simulink subsystem "mesh_assembly"  (R2021a)
settings: Solver=VariableStepAuto  StartTime=0.0  StopTime=10.0  RelTol=1e-3
undefined symbols (not defined in the file): dnm, knm, X, Y, Z
libraries: sm_lib x110, mesh_assembly_library x15
(part 1 of 4)
settings Model: DefaultTestHarness=mechanics_model_measure_transforms  Creator=Daniel Adejumo  LastModifiedBy=Daniel Adejumo

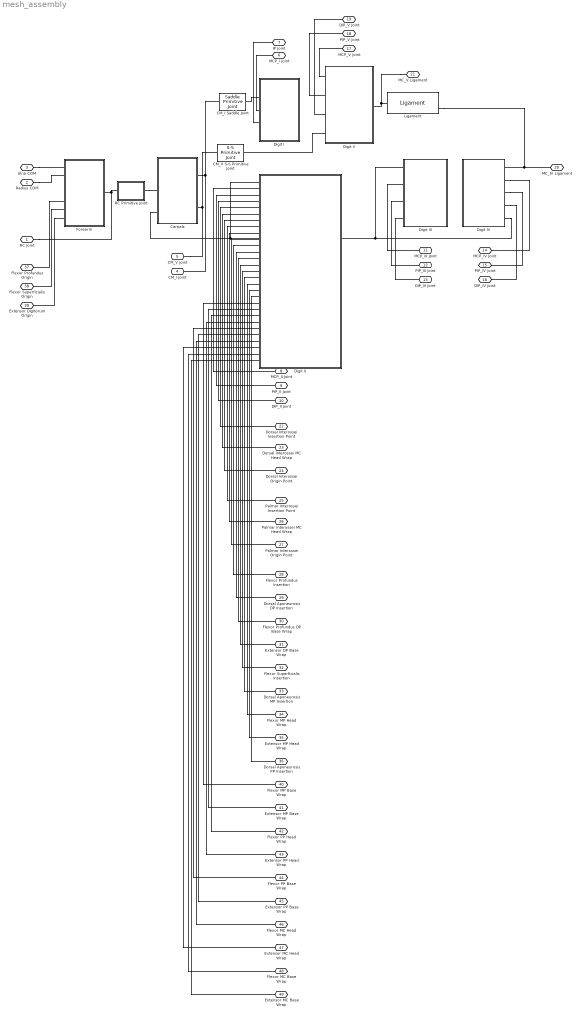
== system mesh_assembly ==
  CM_I Saddle Joint : mesh_assembly_library/Saddle Primitive Joint  stiffness=0  damping=0  x_limits=[-90 90]  y_limits=[-90 90]  z_limits=[-90 90]  x_initial_position=0  y_initial_position=0  z_initial_position=0  centre_block_dim=knm.carpals.cm_i_joint_centre_block_dim  centre_block_density=0  thickness=viz.carpals.cm_1_joint.thickness  x_radius=viz.carpals.cm_1_joint.x_radius  x_length=viz.carpals.cm_1_joint.x_length  x_color=viz.carpals.cm_1_joint.x_color  x_opacity=viz.carpals.cm_1_joint.x_opacity  y_radius=viz.carpals.cm_1_joint.y_radius  y_length=viz.carpals.cm_1_joint.y_length  y_color=viz.carpals.cm_1_joint.y_color  y_opacity=viz.carpals.cm_1_joint.y_opacity  z_radius=viz.carpals.cm_1_joint.z_radius  z_length=viz.carpals.cm_1_joint.z_length  z_color=viz.carpals.cm_1_joint.z_color  z_opacity=viz.carpals.cm_1_joint.z_opacity
  CM_V S-S Primitive Joint : mesh_assembly_library/S-S Primitive Joint  stiffness=0  damping=0  x_limits=[-90 90]  y_limits=[-90 90]  x_initial_position=0  y_initial_position=0  radius=viz.carpals.cm_v_joint.radius  color=viz.carpals.cm_v_joint.color  opacity=viz.carpals.cm_v_joint.opacity
  Carpals : Subsystem
  Digit I : Subsystem
  Digit II : Subsystem
  Digit III : Subsystem
  Digit IV : Subsystem
  Digit V : Subsystem
  Forearm : Subsystem
  Ligament : mesh_assembly_library/Ligament  length=knm.d5.metacarpal_head_ligament.length  width=knm.d5.metacarpal_head_ligament.width  thickness=knm.d5.metacarpal_head_ligament.thickness  tension_stiffness=35E3  tension_damping_coefficient=100  transition_region_width=1e-3  density=800  damping_coefficient=0.2
  RC Primitive Joint : Subsystem  AncestorBlock=mechanics_model_library/S-S Primitive Joint  mask{stiffness=0, damping=0, x_limits=[-90 90], y_limits=[-90 90], x_initial_position=0, y_initial_position=0, thickness=viz.forearm.rc_joint.thickness, x_radius=viz.forearm.rc_joint.x_radius, x_length=viz.forearm.rc_joint.x_length, x_color=viz.forearm.rc_joint.x_color, x_opacity=viz.forearm.rc_joint.x_opacity, y_radius=viz.forearm.rc_joint.y_radius, y_length=viz.forearm.rc_joint.y_length, y_color=viz.forearm.rc_joint.y_color, y_opacity=viz.forearm.rc_joint.y_opacity}
      mask prompts: x_limits "X Limits"; y_limits "Y Limits"; x_initial_position "X Initial Position"; y_initial_position "Y Initial Position"; thickness "Thickness [m]"; x_radius "X Radius [m]"; x_length "X Length [m]"; x_color "X Color (RGB - Range [0, 1])"; x_opacity "X Opacity (Range [0, 1])"; y_radius "Y Radius [m]"; y_length "Y Length [m]"; y_color "Y Color (RGB - Range [0, 1])"; y_opacity "Y Opacity (Range [0, 1])"
      mask DialogControl DescGroupVar Prompt: Radiocarpal Primitive Joint
      mask DialogControl DescTextVar Prompt: Primitive representation of the radiocarpal joint using a universal joint. This is found at the Radiocarpal joint.
      mask DialogControl Container4 Prompt: Mechanics
      mask DialogControl Container6 Prompt: Visualization
      mask DialogControl Container7 Prompt: X Axis
      mask DialogControl Container8 Prompt: Y Axis
  RC Joint : PMIOPort  Side=Left
  Radius COM : PMIOPort  Port=2  Side=Left
  Ulna COM : PMIOPort  Port=3  Side=Left
  CM_I Joint : PMIOPort  Port=4  Side=Left
  CM_V Joint : PMIOPort  Port=5  Side=Left
  MCP_I Joint : PMIOPort  Port=6  Side=Left
  IP Joint : PMIOPort  Port=7  Side=Left
  MCP_II Joint : PMIOPort  Port=8  Side=Left
  PIP_II Joint : PMIOPort  Port=9  Side=Left
  DIP_II Joint : PMIOPort  Port=10  Side=Left
  MCP_III Joint : PMIOPort  Port=11  Side=Left
  PIP_III Joint : PMIOPort  Port=12  Side=Left
  DIP_III Joint : PMIOPort  Port=13  Side=Left
  MCP_IV Joint : PMIOPort  Port=14  Side=Left
  PIP_IV Joint : PMIOPort  Port=15  Side=Left
  DIP_IV Joint : PMIOPort  Port=16  Side=Left
  MCP_V Joint : PMIOPort  Port=17  Side=Left
  PIP_V Joint : PMIOPort  Port=18  Side=Left
  DIP_V Joint : PMIOPort  Port=19  Side=Left
  MC_IV Ligament : PMIOPort  Port=20  Side=Right
  MC_V Ligament : PMIOPort  Port=21  Side=Right
  Dorsal Interossei Insertion Point : PMIOPort  Port=22  Side=Left
  Dorsal Interossei MC Head Wrap : PMIOPort  Port=23  Side=Left
  Dorsal Interossei Origin Point : PMIOPort  Port=24  Side=Left
  Palmar Interossei Insertion Point : PMIOPort  Port=25  Side=Left
  Palmar Interossei MC Head Wrap : PMIOPort  Port=26  Side=Left
  Palmar Interossei Origin Point : PMIOPort  Port=27  Side=Left
  Flexor Profundus Insertion : PMIOPort  Port=28  Side=Left
  Dorsal Aponeurosis DP Insertion : PMIOPort  Port=29  Side=Left
  Flexor Profundus DP Base Wrap : PMIOPort  Port=30  Side=Left
  Extensor DP Base Wrap : PMIOPort  Port=31  Side=Left
  Flexor Superficialis Insertion : PMIOPort  Port=32  Side=Left
  Dorsal Aponeurosis MP Insertion : PMIOPort  Port=33  Side=Left
  Flexor MP Head Wrap : PMIOPort  Port=34  Side=Left
  Extensor MP Head Wrap : PMIOPort  Port=35  Side=Left
  Dorsal Aponeurosis PP Insertion : PMIOPort  Port=36  Side=Left
  Flexor Profundus Origin : PMIOPort  Port=37  Side=Left
  Flexor Superficialis Origin : PMIOPort  Port=38  Side=Left
  Extensor Digitorum Origin : PMIOPort  Port=39  Side=Left
  Flexor MP Base Wrap : PMIOPort  Port=40  Side=Left
  Extensor MP Base Wrap : PMIOPort  Port=41  Side=Left
  Flexor PP Head Wrap : PMIOPort  Port=42  Side=Left
  Extensor PP Head Wrap : PMIOPort  Port=43  Side=Left
  Flexor PP Base Wrap : PMIOPort  Port=44  Side=Left
  Extensor PP Base Wrap : PMIOPort  Port=45  Side=Left
  Flexor MC Head Wrap : PMIOPort  Port=46  Side=Left
  Extensor MC Head Wrap : PMIOPort  Port=47  Side=Left
  Flexor MC Base Wrap : PMIOPort  Port=48  Side=Left
  Extensor MC Base Wrap : PMIOPort  Port=49  Side=Left
  connections:
  RC Primitive Joint/LConn1 -- Forearm/RConn1 -- RC Joint/RConn1
  Digit IV/LConn5 -- Digit III/LConn1 -- Digit II/LConn1 -- Carpals/LConn3
  CM_I Joint/RConn1 -- Carpals/RConn1 -- CM_I Saddle Joint/LConn1
  MC_V Ligament/RConn1 -- Ligament/LConn1 -- Digit V/RConn1
  CM_V Joint/RConn1 -- Carpals/RConn2 -- CM_V S-S Primitive Joint/LConn1
  MC_IV Ligament/RConn1 -- Ligament/RConn1 -- Digit IV/LConn1
  Digit V/LConn4 -- CM_V S-S Primitive Joint/RConn1
  Digit I/LConn2 -- CM_I Saddle Joint/RConn1
  Radius COM/RConn1 -- Forearm/LConn2
  Ulna COM/RConn1 -- Forearm/LConn1
  MCP_I Joint/RConn1 -- Digit I/LConn3
  IP Joint/RConn1 -- Digit I/LConn4
  Digit II/LConn2 -- MCP_II Joint/RConn1
  Digit II/LConn3 -- PIP_II Joint/RConn1
  Digit II/LConn4 -- DIP_II Joint/RConn1
  Digit III/LConn4 -- DIP_III Joint/RConn1
  Digit III/LConn3 -- PIP_III Joint/RConn1
  Digit III/LConn2 -- MCP_III Joint/RConn1
  Digit IV/LConn2 -- MCP_IV Joint/RConn1
  Digit IV/LConn3 -- PIP_IV Joint/RConn1
  Digit IV/LConn4 -- DIP_IV Joint/RConn1
  PIP_V Joint/RConn1 -- Digit V/LConn2
  Digit V/LConn3 -- DIP_V Joint/RConn1
  MCP_V Joint/RConn1 -- Digit V/LConn1
  RC Primitive Joint/RConn1 -- Carpals/LConn2
  Digit II/LConn5 -- Dorsal Interossei Insertion Point/RConn1
  Digit II/LConn6 -- Dorsal Interossei MC Head Wrap/RConn1
  Digit II/LConn7 -- Dorsal Interossei Origin Point/RConn1
  Digit II/LConn8 -- Palmar Interossei Insertion Point/RConn1
  Digit II/LConn9 -- Palmar Interossei MC Head Wrap/RConn1
  Digit II/LConn10 -- Palmar Interossei Origin Point/RConn1
  Digit II/LConn11 -- Flexor Profundus Insertion/RConn1
  Digit II/LConn12 -- Dorsal Aponeurosis DP Insertion/RConn1
  Digit II/LConn13 -- Flexor Profundus DP Base Wrap/RConn1
  Digit II/LConn14 -- Extensor DP Base Wrap/RConn1
  Digit II/LConn15 -- Flexor Superficialis Insertion/RConn1
  Digit II/LConn16 -- Dorsal Aponeurosis MP Insertion/RConn1
  Digit II/LConn17 -- Flexor MP Head Wrap/RConn1
  Digit II/LConn18 -- Extensor MP Head Wrap/RConn1
  Digit II/LConn19 -- Dorsal Aponeurosis PP Insertion/RConn1
  Forearm/LConn5 -- Flexor Profundus Origin/RConn1
  Forearm/LConn6 -- Flexor Superficialis Origin/RConn1
  Forearm/LConn7 -- Extensor Digitorum Origin/RConn1
  Digit II/LConn20 -- Flexor MP Base Wrap/RConn1
  Digit II/LConn21 -- Extensor MP Base Wrap/RConn1
  Digit II/LConn22 -- Flexor PP Head Wrap/RConn1
  Digit II/LConn23 -- Extensor PP Head Wrap/RConn1
  Digit II/LConn24 -- Flexor PP Base Wrap/RConn1
  Digit II/LConn25 -- Extensor PP Base Wrap/RConn1
  Digit II/LConn26 -- Flexor MC Head Wrap/RConn1
  Digit II/LConn27 -- Extensor MC Head Wrap/RConn1
  Digit II/LConn28 -- Flexor MC Base Wrap/RConn1
  Digit II/LConn29 -- Extensor MC Base Wrap/RConn1

== system mesh_assembly/Carpals ==
  CM_I Joint Transform : sm_lib/Frames and Transforms/Rigid Transform  TranslationMethod=Cartesian  TranslationStandardOffset=0  TranslationLengthUnit=m  TranslationStandardAxis=+Z  TranslationCartesianOffset=knm.carpals.cm_i_joint_transform(1, :)  TranslationROffset=0  TranslationROffsetUnits=m  TranslationZOffset=0  TranslationZOffsetUnits=m  TranslationThetaOffset=0  TranslationThetaOffsetUnits=deg  RotationMethod=RotationSequence  RotationAngleUnits=deg  RotationStandardAxis=+Z  RotationAngle=0.0  RotationArbitraryAxis=[0 0 1]  FollAlignAxisA=+X  BaseAlignAxisA=+Y  FollAlignAxisB=+Y  BaseAlignAxisB=+Z  RotationSequenceAxes=FollowerAxes  RotationSequence=XYZ  RotationSequenceAngles=knm.carpals.cm_i_joint_transform(2, :)  RotationSequenceAnglesUnits=deg  RotationMatrix=[1 0 0; 0 1 0; 0 0 1]
  CM_V Joint Transform : sm_lib/Frames and Transforms/Rigid Transform  TranslationMethod=Cartesian  TranslationStandardOffset=0  TranslationLengthUnit=m  TranslationStandardAxis=+Z  TranslationCartesianOffset=knm.carpals.cm_v_joint_transform(1, :)  TranslationROffset=0  TranslationROffsetUnits=m  TranslationZOffset=0  TranslationZOffsetUnits=m  TranslationThetaOffset=0  TranslationThetaOffsetUnits=deg  RotationMethod=RotationSequence  RotationAngleUnits=deg  RotationStandardAxis=+Z  RotationAngle=0.0  RotationArbitraryAxis=[0 0 1]  FollAlignAxisA=+X  BaseAlignAxisA=+Y  FollAlignAxisB=+Y  BaseAlignAxisB=+Z  RotationSequenceAxes=FollowerAxes  RotationSequence=XYZ  RotationSequenceAngles=knm.carpals.cm_v_joint_transform(2, :)  RotationSequenceAnglesUnits=deg  RotationMatrix=[1 0 0; 0 1 0; 0 0 1]
  Carpals : sm_lib/Body Elements/File Solid  ExtGeomFileName=C:\Users\Daniel Adejumo\Documents\MATLAB\DARM\Geometry Models and FEA\Models\Skeleton Scan\Right Hand\Carpals.obj  UnitType=Custom  ExtGeomFileUnits=mm  StepReaderType=HEX  ExportConvexHullGeometry=off  InertiaType=CalculateFromGeometry  Mass=1  MassUnits=kg  CenterOfMass=[0 0 0]  CenterOfMassUnits=m  MomentsOfInertia=[1 1 1]  MomentsOfInertiaUnits=kg*m^2  ProductsOfInertia=[0 0 0]  ProductsOfInertiaUnits=kg*m^2  BasedOnType=Density  Density=dnm.link_density  DensityUnits=kg/m^3  DoExposeReferenceFrame=on  SerializedFrames=<Frames><Frame><Id>Frame1</Id><Value><Name>COM</Name><Origin><Source>CenterOfMassFrame</Source><FeatureName></FeatureName></Origin><PrimaryAxis><DefinedDirection>+Z</DefinedDirection><Source>ReferenceFrame</Source><SourceDirection>-Z</SourceDirection><FeatureName></FeatureName></PrimaryAxis><SecondaryAxis><DefinedDirection>+X</DefinedDirection><Source>ReferenceFrame</Source><SourceDirection>-Y</SourceDirection><FeatureName></FeatureName></SecondaryAxis></Value></Frame></Frames>  GraphicType=FromGeometry  MarkerShape=Sphere  MarkerSize=10  GraphicVisPropType=SimpleVisualProperties  GraphicDiffuseColor=[0.5 0.5 0.5]  GraphicSpecularColor=[0.5 0.5 0.5 1.0]  GraphicAmbientColor=[0.15 0.15 0.15 1.0]  GraphicEmissiveColor=[0.0 0.0 0.0 1.0]  GraphicShininess=75  GraphicOpacity=1.0
  RC Joint Transform : sm_lib/Frames and Transforms/Rigid Transform  TranslationMethod=Cartesian  TranslationStandardOffset=0  TranslationLengthUnit=m  TranslationStandardAxis=+Z  TranslationCartesianOffset=knm.carpals.rc_joint_transform(1, :)  TranslationROffset=0  TranslationROffsetUnits=m  TranslationZOffset=0  TranslationZOffsetUnits=m  TranslationThetaOffset=0  TranslationThetaOffsetUnits=deg  RotationMethod=RotationSequence  RotationAngleUnits=deg  RotationStandardAxis=+Z  RotationAngle=0.0  RotationArbitraryAxis=[0 0 1]  FollAlignAxisA=+X  BaseAlignAxisA=+Y  FollAlignAxisB=+Y  BaseAlignAxisB=+Z  RotationSequenceAxes=FollowerAxes  RotationSequence=XYZ  RotationSequenceAngles=knm.carpals.rc_joint_transform(2, :)  RotationSequenceAnglesUnits=deg  RotationMatrix=[1 0 0; 0 1 0; 0 0 1]
  Carpals COM : PMIOPort  Side=Left
  RC Joint : PMIOPort  Port=2  Side=Left
  Carpals R : PMIOPort  Port=3  Side=Left
  CM_I Joint : PMIOPort  Port=4  Side=Right
  CM_V Joint : PMIOPort  Port=5  Side=Right
  connections:
  CM_V Joint/RConn1 -- CM_V Joint Transform/RConn1
  CM_I Joint/RConn1 -- CM_I Joint Transform/RConn1
  Carpals R/RConn1 -- Carpals/RConn1
  CM_I Joint Transform/LConn1 -- Carpals/LConn1 -- CM_V Joint Transform/LConn1 -- RC Joint Transform/LConn1 -- Carpals COM/RConn1
  RC Joint/RConn1 -- RC Joint Transform/RConn1

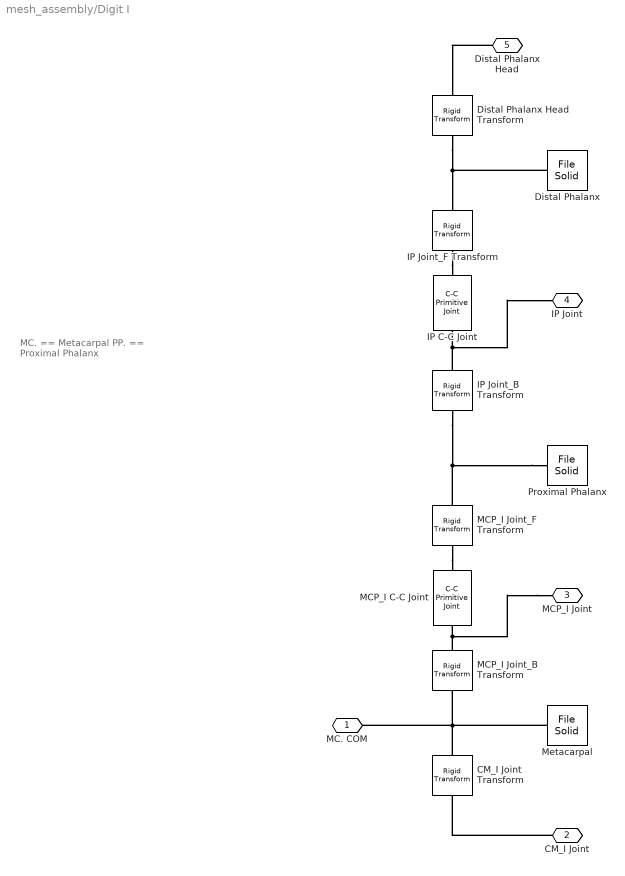
== system mesh_assembly/Digit I ==
  note: MC. == Metacarpal
      | PP. == Proximal Phalanx
  CM_I Joint Transform : sm_lib/Frames and Transforms/Rigid Transform  TranslationMethod=Cartesian  TranslationStandardOffset=0  TranslationLengthUnit=m  TranslationStandardAxis=+Z  TranslationCartesianOffset=knm.d1.metacarpal.cm_joint_transform(1, :)  TranslationROffset=0  TranslationROffsetUnits=m  TranslationZOffset=0  TranslationZOffsetUnits=m  TranslationThetaOffset=0  TranslationThetaOffsetUnits=deg  RotationMethod=RotationSequence  RotationAngleUnits=deg  RotationStandardAxis=+Z  RotationAngle=0.0  RotationArbitraryAxis=[0 0 1]  FollAlignAxisA=+X  BaseAlignAxisA=+Y  FollAlignAxisB=+Y  BaseAlignAxisB=+Z  RotationSequenceAxes=FollowerAxes  RotationSequence=XYZ  RotationSequenceAngles=knm.d1.metacarpal.cm_joint_transform(2, :)  RotationSequenceAnglesUnits=deg  RotationMatrix=[1 0 0; 0 1 0; 0 0 1]
  Distal Phalanx : sm_lib/Body Elements/File Solid  ExtGeomFileName=C:\Users\Daniel Adejumo\Documents\MATLAB\DARM\Geometry Models and FEA\Models\Skeleton Scan\Right Hand\Digit I\Distal Phalanx I.obj  UnitType=Custom  ExtGeomFileUnits=in  StepReaderType=HEX  ExportConvexHullGeometry=off  InertiaType=CalculateFromGeometry  Mass=1  MassUnits=kg  CenterOfMass=[0 0 0]  CenterOfMassUnits=m  MomentsOfInertia=[1 1 1]  MomentsOfInertiaUnits=kg*m^2  ProductsOfInertia=[0 0 0]  ProductsOfInertiaUnits=kg*m^2  BasedOnType=Density  Density=dnm.link_density  DensityUnits=kg/m^3  DoExposeReferenceFrame=on  SerializedFrames=<Frames><Frame><Id>Frame1</Id><Value><Name>COM</Name><Origin><Source>CenterOfMassFrame</Source><FeatureName></FeatureName></Origin><PrimaryAxis><DefinedDirection>+Z</DefinedDirection><Source>ReferenceFrame</Source><SourceDirection>-Z</SourceDirection><FeatureName></FeatureName></PrimaryAxis><SecondaryAxis><DefinedDirection>+X</DefinedDirection><Source>ReferenceFrame</Source><SourceDirection>+X</SourceDirection><FeatureName></FeatureName></SecondaryAxis></Value></Frame></Frames>  GraphicType=FromGeometry  MarkerShape=Sphere  MarkerSize=10  GraphicVisPropType=SimpleVisualProperties  GraphicDiffuseColor=[0.5 0.5 0.5]  GraphicSpecularColor=[0.5 0.5 0.5 1.0]  GraphicAmbientColor=[0.15 0.15 0.15 1.0]  GraphicEmissiveColor=[0.0 0.0 0.0 1.0]  GraphicShininess=75  GraphicOpacity=1.0
  Distal Phalanx Head Transform : sm_lib/Frames and Transforms/Rigid Transform  TranslationMethod=Cartesian  TranslationStandardOffset=0  TranslationLengthUnit=m  TranslationStandardAxis=+Z  TranslationCartesianOffset=knm.d1.distal_phalanx.head_transform(1, :)  TranslationROffset=0  TranslationROffsetUnits=m  TranslationZOffset=0  TranslationZOffsetUnits=m  TranslationThetaOffset=0  TranslationThetaOffsetUnits=deg  RotationMethod=RotationSequence  RotationAngleUnits=deg  RotationStandardAxis=+Z  RotationAngle=0.0  RotationArbitraryAxis=[0 0 1]  FollAlignAxisA=+X  BaseAlignAxisA=+Y  FollAlignAxisB=+Y  BaseAlignAxisB=+Z  RotationSequenceAxes=FollowerAxes  RotationSequence=XYZ  RotationSequenceAngles=knm.d1.distal_phalanx.head_transform(2, :)  RotationSequenceAnglesUnits=deg  RotationMatrix=[1 0 0; 0 1 0; 0 0 1]
  IP C-C Joint : mesh_assembly_library/C-C Primitive Joint  stiffness=0  damping=0  lower_limit=-90  upper_limit=90  initial_position=0  radius=viz.d1.ip_joint.radius  length=viz.d1.ip_joint.length  thickness=viz.d1.ip_joint.thickness  color=viz.d1.ip_joint.color  opacity=viz.d1.ip_joint.opacity
  IP Joint_B Transform : sm_lib/Frames and Transforms/Rigid Transform  TranslationMethod=Cartesian  TranslationStandardOffset=0  TranslationLengthUnit=m  TranslationStandardAxis=+Z  TranslationCartesianOffset=knm.d1.proximal_phalanx.ip_joint_transform(1, :)  TranslationROffset=0  TranslationROffsetUnits=m  TranslationZOffset=0  TranslationZOffsetUnits=m  TranslationThetaOffset=0  TranslationThetaOffsetUnits=deg  RotationMethod=RotationSequence  RotationAngleUnits=deg  RotationStandardAxis=+Z  RotationAngle=0.0  RotationArbitraryAxis=[0 0 1]  FollAlignAxisA=+X  BaseAlignAxisA=+Y  FollAlignAxisB=+Y  BaseAlignAxisB=+Z  RotationSequenceAxes=FollowerAxes  RotationSequence=XYZ  RotationSequenceAngles=knm.d1.proximal_phalanx.ip_joint_transform(2, :)  RotationSequenceAnglesUnits=deg  RotationMatrix=[1 0 0; 0 1 0; 0 0 1]
  IP Joint_F Transform : sm_lib/Frames and Transforms/Rigid Transform  TranslationMethod=Cartesian  TranslationStandardOffset=0  TranslationLengthUnit=m  TranslationStandardAxis=+Z  TranslationCartesianOffset=knm.d1.distal_phalanx.ip_joint_transform(1, :)  TranslationROffset=0  TranslationROffsetUnits=m  TranslationZOffset=0  TranslationZOffsetUnits=m  TranslationThetaOffset=0  TranslationThetaOffsetUnits=deg  RotationMethod=RotationSequence  RotationAngleUnits=deg  RotationStandardAxis=+Z  RotationAngle=0.0  RotationArbitraryAxis=[0 0 1]  FollAlignAxisA=+X  BaseAlignAxisA=+Y  FollAlignAxisB=+Y  BaseAlignAxisB=+Z  RotationSequenceAxes=FollowerAxes  RotationSequence=XYZ  RotationSequenceAngles=knm.d1.distal_phalanx.ip_joint_transform(2, :)  RotationSequenceAnglesUnits=deg  RotationMatrix=[1 0 0; 0 1 0; 0 0 1]
  MCP_I C-C Joint : mesh_assembly_library/C-C Primitive Joint  stiffness=0  damping=0  lower_limit=-90  upper_limit=90  initial_position=0  radius=viz.d1.mcp_joint.radius  length=viz.d1.mcp_joint.length  thickness=viz.d1.mcp_joint.thickness  color=viz.d1.mcp_joint.color  opacity=viz.d1.mcp_joint.opacity
  MCP_I Joint_B Transform : sm_lib/Frames and Transforms/Rigid Transform  TranslationMethod=Cartesian  TranslationStandardOffset=0  TranslationLengthUnit=m  TranslationStandardAxis=+Z  TranslationCartesianOffset=knm.d1.metacarpal.mcp_joint_transform(1, :)  TranslationROffset=0  TranslationROffsetUnits=m  TranslationZOffset=0  TranslationZOffsetUnits=m  TranslationThetaOffset=0  TranslationThetaOffsetUnits=deg  RotationMethod=RotationSequence  RotationAngleUnits=deg  RotationStandardAxis=+Z  RotationAngle=0.0  RotationArbitraryAxis=[0 0 1]  FollAlignAxisA=+X  BaseAlignAxisA=+Y  FollAlignAxisB=+Y  BaseAlignAxisB=+Z  RotationSequenceAxes=FollowerAxes  RotationSequence=XYZ  RotationSequenceAngles=knm.d1.metacarpal.mcp_joint_transform(2, :)  RotationSequenceAnglesUnits=deg  RotationMatrix=[1 0 0; 0 1 0; 0 0 1]
  MCP_I Joint_F Transform : sm_lib/Frames and Transforms/Rigid Transform  TranslationMethod=Cartesian  TranslationStandardOffset=0  TranslationLengthUnit=m  TranslationStandardAxis=+Z  TranslationCartesianOffset=knm.d1.proximal_phalanx.mcp_joint_transform(1, :)  TranslationROffset=0  TranslationROffsetUnits=m  TranslationZOffset=0  TranslationZOffsetUnits=m  TranslationThetaOffset=0  TranslationThetaOffsetUnits=deg  RotationMethod=RotationSequence  RotationAngleUnits=deg  RotationStandardAxis=+Z  RotationAngle=0.0  RotationArbitraryAxis=[0 0 1]  FollAlignAxisA=+X  BaseAlignAxisA=+Y  FollAlignAxisB=+Y  BaseAlignAxisB=+Z  RotationSequenceAxes=FollowerAxes  RotationSequence=XYZ  RotationSequenceAngles=knm.d1.proximal_phalanx.mcp_joint_transform(2, :)  RotationSequenceAnglesUnits=deg  RotationMatrix=[1 0 0; 0 1 0; 0 0 1]
  Metacarpal : sm_lib/Body Elements/File Solid  ExtGeomFileName=C:\Users\Daniel Adejumo\Documents\MATLAB\DARM\Geometry Models and FEA\Models\Skeleton Scan\Right Hand\Digit I\Metacarpal I.obj  UnitType=Custom  ExtGeomFileUnits=mm  StepReaderType=HEX  ExportConvexHullGeometry=off  InertiaType=CalculateFromGeometry  Mass=1  MassUnits=kg  CenterOfMass=[0 0 0]  CenterOfMassUnits=m  MomentsOfInertia=[1 1 1]  MomentsOfInertiaUnits=kg*m^2  ProductsOfInertia=[0 0 0]  ProductsOfInertiaUnits=kg*m^2  BasedOnType=Density  Density=dnm.link_density  DensityUnits=kg/m^3  DoExposeReferenceFrame=on  SerializedFrames=<Frames><Frame><Id>Frame1</Id><Value><Name>COM</Name><Origin><Source>CenterOfMassFrame</Source><FeatureName></FeatureName></Origin><PrimaryAxis><DefinedDirection>+Z</DefinedDirection><Source>ReferenceFrame</Source><SourceDirection>-Z</SourceDirection><FeatureName></FeatureName></PrimaryAxis><SecondaryAxis><DefinedDirection>+X</DefinedDirection><Source>ReferenceFrame</Source><SourceDirection>+X</SourceDirection><FeatureName></FeatureName></SecondaryAxis></Value></Frame></Frames>  GraphicType=FromGeometry  MarkerShape=Sphere  MarkerSize=10  GraphicVisPropType=SimpleVisualProperties  GraphicDiffuseColor=[0.5 0.5 0.5]  GraphicSpecularColor=[0.5 0.5 0.5 1.0]  GraphicAmbientColor=[0.15 0.15 0.15 1.0]  GraphicEmissiveColor=[0.0 0.0 0.0 1.0]  GraphicShininess=75  GraphicOpacity=1.0
  Proximal Phalanx : sm_lib/Body Elements/File Solid  ExtGeomFileName=C:\Users\Daniel Adejumo\Documents\MATLAB\DARM\Geometry Models and FEA\Models\Skeleton Scan\Right Hand\Digit I\Proximal Phalanx I.obj  UnitType=Custom  ExtGeomFileUnits=mm  StepReaderType=HEX  ExportConvexHullGeometry=off  InertiaType=CalculateFromGeometry  Mass=1  MassUnits=kg  CenterOfMass=[0 0 0]  CenterOfMassUnits=m  MomentsOfInertia=[1 1 1]  MomentsOfInertiaUnits=kg*m^2  ProductsOfInertia=[0 0 0]  ProductsOfInertiaUnits=kg*m^2  BasedOnType=Density  Density=dnm.link_density  DensityUnits=kg/m^3  DoExposeReferenceFrame=on  SerializedFrames=<Frames><Frame><Id>Frame1</Id><Value><Name>COM</Name><Origin><Source>CenterOfMassFrame</Source><FeatureName></FeatureName></Origin><PrimaryAxis><DefinedDirection>+Z</DefinedDirection><Source>ReferenceFrame</Source><SourceDirection>-Z</SourceDirection><FeatureName></FeatureName></PrimaryAxis><SecondaryAxis><DefinedDirection>+X</DefinedDirection><Source>ReferenceFrame</Source><SourceDirection>+X</SourceDirection><FeatureName></FeatureName></SecondaryAxis></Value></Frame></Frames>  GraphicType=FromGeometry  MarkerShape=Sphere  MarkerSize=10  GraphicVisPropType=SimpleVisualProperties  GraphicDiffuseColor=[0.5 0.5 0.5]  GraphicSpecularColor=[0.5 0.5 0.5 1.0]  GraphicAmbientColor=[0.15 0.15 0.15 1.0]  GraphicEmissiveColor=[0.0 0.0 0.0 1.0]  GraphicShininess=75  GraphicOpacity=1.0
  MC. COM : PMIOPort  Side=Left
  CM_I Joint : PMIOPort  Port=2  Side=Left
  MCP_I Joint : PMIOPort  Port=3  Side=Left
  IP Joint : PMIOPort  Port=4  Side=Left
  Distal Phalanx Head : PMIOPort  Port=5  Side=Left
  connections:
  Distal Phalanx Head/RConn1 -- Distal Phalanx Head Transform/RConn1
  IP Joint_F Transform/RConn1 -- IP C-C Joint/RConn1
  IP C-C Joint/LConn1 -- IP Joint/RConn1 -- IP Joint_B Transform/RConn1
  Distal Phalanx Head Transform/LConn1 -- Distal Phalanx/LConn1 -- IP Joint_F Transform/LConn1
  MCP_I Joint/RConn1 -- MCP_I Joint_B Transform/RConn1 -- MCP_I C-C Joint/LConn1
  MCP_I Joint_F Transform/RConn1 -- MCP_I C-C Joint/RConn1
  Proximal Phalanx/LConn1 -- IP Joint_B Transform/LConn1 -- MCP_I Joint_F Transform/LConn1
  CM_I Joint/RConn1 -- CM_I Joint Transform/RConn1
  MCP_I Joint_B Transform/LConn1 -- MC. COM/RConn1 -- CM_I Joint Transform/LConn1 -- Metacarpal/LConn1
